simulink model "BrakeCtrl_V1"  (R2018a)
settings: Solver=VariableStepAuto  StartTime=0.0  StopTime=10.0  FixedStep=sampletime  RelTol=1e-3  EnableMultiTasking=on
PreLoadFcn:
  | BrakeCtrl_V1_PreLoad
values from neighbouring files (symbols this model uses):
  DrvReqBrkTrqMax_K = 500    [BrakeCtrl_V1_PreLoad.m]
  RegnBrkFct_K = 1.0    (= 1)    [BrakeCtrl_V1_PreLoad.m]
libraries: simulink x2
settings Model: Creator=IAEC nishito  LastModifiedBy=nishito
settings DataIOCC: LimitDataPoints=on  SaveFormat=Array  SignalLoggingSaveFormat=ModelDataLogs  SaveOutput=off  SaveTime=off
settings OptimizationCC: DefaultParameterBehavior=Inlined  ExpressionDepthLimit=2147483647  LifeSpan=inf
settings DebuggingCC: UnderspecifiedInitializationDetection=Classic  MergeDetectMultiDrivingBlocksExec=none  SolverPrmCheckMsg=warning  FcnCallInpInsideContextMsg=warning  StateNameClashWarn=warning  SFUnexpectedBacktrackingDiag=warning  SFNoUnconditionalDefaultTransitionDiag=warning  SFExecutionAtInitializationDiag=none
settings HardwareCC: ProdBitPerPointer=32  ProdBitPerSizeT=32  ProdBitPerPtrDiffT=32  ProdLargestAtomicFloat=None  ProdIntDivRoundTo=Undefined  ProdEndianess=Unspecified  ProdWordSize=32  ProdHWDeviceType=32-bit Generic
settings ModelReferenceCC: UpdateModelReferenceTargets=IfOutOfDate  PropagateSignalLabelsOutOfModel=off
settings CodeAppCC: StateflowObjectComments=on
settings GRTTargetCC: TargetLangStandard=C89/C90 (ANSI)  GeneratePreprocessorConditionals=Disable all  CombineOutputUpdateFcns=off  GRTInterface=on
settings ConfigComp: CovMetricSettings=dw  CovHtmlReporting=on  CovSaveCumulativeToWorkspaceVar=on  CovSaveSingleToWorkspaceVar=on  CovExternalEMLEnable=off

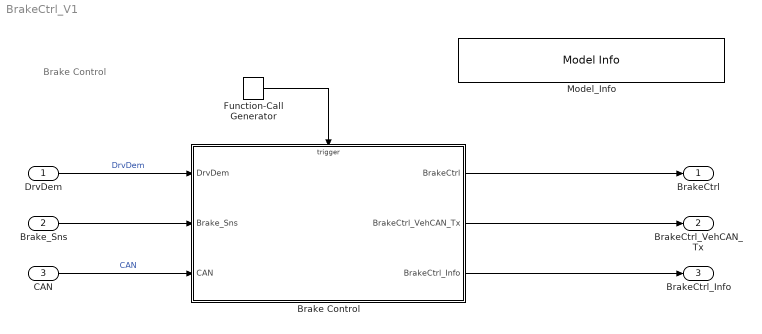
== system BrakeCtrl_V1 ==
  note: Brake Control
  DrvDem : Inport  OutDataTypeStr=Bus: Driver_demand_Bus
      settings: AttributesFormatString=%<OutDataTypeStr>
  Brake_Sns : Inport  Port=2  OutDataTypeStr=Bus: Brake_sensor_Bus
      settings: AttributesFormatString=%<OutDataTypeStr>
  CAN : Inport  Port=3  OutDataTypeStr=Bus: CAN_Bus
      settings: AttributesFormatString=<%<OutDataTypeStr>>
  Brake Control : Subsystem
  Function-Call Generator : simulink/Ports & Subsystems/Function-Call Generator  sample_time=0.01  numberOfIterations=1
      settings: AttributesFormatString=<sample_time=%<sample_time>>
  Model_Info : simulink/Model-Wide Utilities/Model Info  Frame=on  DisplayStringWithTags=|  HorizontalTextAlignment=Left  LeftAlignmentValue=0.02
      | Version  %<ModelVersion>
      | LastModifided by %<LastModifiedBy>  Date %<LastModificationDate>
      | Description  %<Description>
  BrakeCtrl : Outport  OutDataTypeStr=Bus: BrakeCtrl_Bus
      settings: AttributesFormatString=<%<OutDataTypeStr>>
  BrakeCtrl_VehCAN_Tx : Outport  Port=2  OutDataTypeStr=Bus: BrakeCtrl_VehCAN_Tx_Bus
      settings: AttributesFormatString=<%<OutDataTypeStr>>
  BrakeCtrl_Info : Outport  Port=3  OutDataTypeStr=Bus: BrakeCtrl_Info_Bus
      settings: AttributesFormatString=<%<OutDataTypeStr>>
  wires:
  CAN/1 -> Brake Control/3(CAN)  "CAN"
  DrvDem/1 -> Brake Control/1(DrvDem)  "DrvDem"
  Brake_Sns/1 -> Brake Control/2(Brake_Sns)
  Function-Call Generator/1 -> Brake Control/Trigger
  Brake Control/2(BrakeCtrl_VehCAN_Tx) -> BrakeCtrl_VehCAN_Tx/1
  Brake Control/1(BrakeCtrl) -> BrakeCtrl/1
  Brake Control/3(BrakeCtrl_Info) -> BrakeCtrl_Info/1

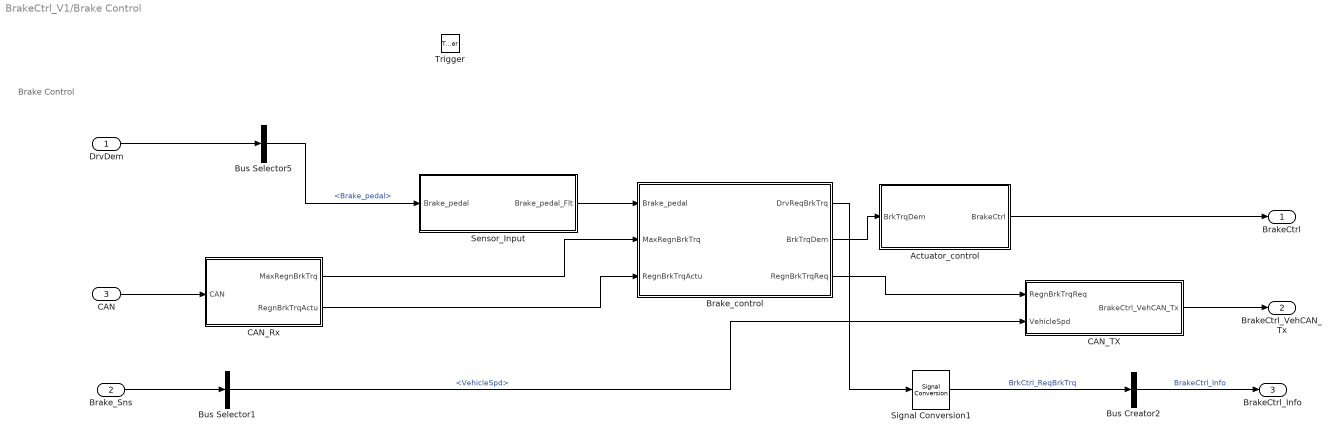
== system BrakeCtrl_V1/Brake Control ==
  note: Brake Control
  DrvDem : Inport
  Brake_Sns : Inport  Port=2
  CAN : Inport  Port=3
  Trigger : TriggerPort  TriggerType=function-call  VariantControl=Variant  PortDimensions=1
  Actuator_control : Subsystem
  Brake_control : Subsystem
  Bus Creator2 : BusCreator  Inputs=1  OutDataTypeStr=Bus: BrakeCtrl_Info_Bus
      settings: AttributesFormatString=%<OutDataTypeStr>
  Bus Selector1 : BusSelector  OutputSignals=VehicleSpd
  Bus Selector5 : BusSelector  OutputSignals=Brake_pedal
  CAN_Rx : Subsystem
  CAN_TX : Subsystem
  Sensor_Input : Subsystem
  Signal Conversion1 : SignalConversion  OverrideOpt=off
  BrakeCtrl : Outport
  BrakeCtrl_VehCAN_Tx : Outport  Port=2
  BrakeCtrl_Info : Outport  Port=3
  wires:
  Brake_Sns/1 -> Bus Selector1/1
  Bus Creator2/1 -> BrakeCtrl_Info/1  "BrakeCtrl_Info"
  Brake_control/3(RegnBrkTrqReq) -> CAN_TX/1(RegnBrkTrqReq)
  CAN_TX/1(BrakeCtrl_VehCAN_Tx) -> BrakeCtrl_VehCAN_Tx/1
  Actuator_control/1(BrakeCtrl) -> BrakeCtrl/1
  Sensor_Input/1(Brake_pedal_Flt) -> Brake_control/1(Brake_pedal)
  Brake_control/2(BrkTrqDem) -> Actuator_control/1(BrkTrqDem)
  DrvDem/1 -> Bus Selector5/1
  Bus Selector5/1 -> Sensor_Input/1(Brake_pedal)  "<Brake_pedal>"
  Bus Selector1/1 -> CAN_TX/2(VehicleSpd)  "<VehicleSpd>"
  Brake_control/1(DrvReqBrkTrq) -> Signal Conversion1/1
  CAN/1 -> CAN_Rx/1(CAN)
  CAN_Rx/1(MaxRegnBrkTrq) -> Brake_control/2(MaxRegnBrkTrq)
  CAN_Rx/2(RegnBrkTrqActu) -> Brake_control/3(RegnBrkTrqActu)
  Signal Conversion1/1 -> Bus Creator2/1  "BrkCtrl_ReqBrkTrq"

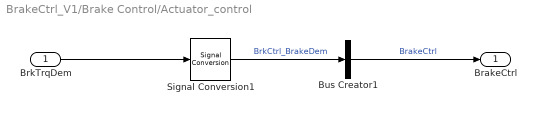
== system BrakeCtrl_V1/Brake Control/Actuator_control ==
  BrkTrqDem : Inport
  Bus Creator1 : BusCreator  Inputs=1  OutDataTypeStr=Bus: BrakeCtrl_Bus
      settings: AttributesFormatString=%<OutDataTypeStr>
  Signal Conversion1 : SignalConversion  OverrideOpt=off
  BrakeCtrl : Outport
  wires:
  Signal Conversion1/1 -> Bus Creator1/1  "BrkCtrl_BrakeDem"
  BrkTrqDem/1 -> Signal Conversion1/1
  Bus Creator1/1 -> BrakeCtrl/1  "BrakeCtrl"

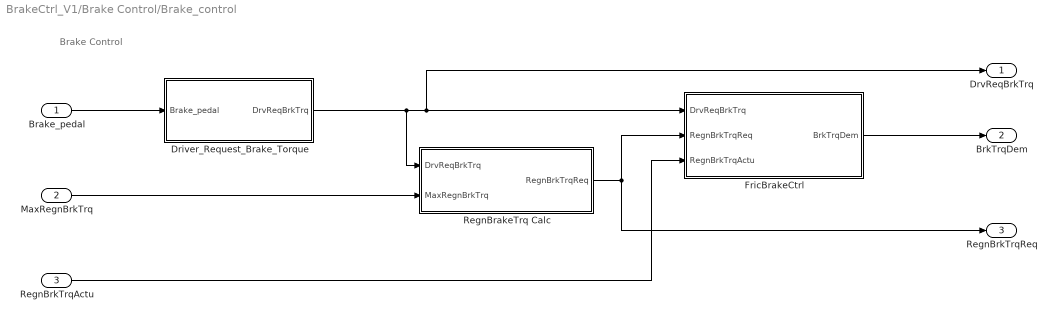
== system BrakeCtrl_V1/Brake Control/Brake_control ==
  note: Brake Control
  Brake_pedal : Inport
  MaxRegnBrkTrq : Inport  Port=2
  RegnBrkTrqActu : Inport  Port=3
  Driver_Request_Brake_Torque : Subsystem
  FricBrakeCtrl : Subsystem
  RegnBrakeTrq Calc : Subsystem
  DrvReqBrkTrq : Outport
  BrkTrqDem : Outport  Port=2
  RegnBrkTrqReq : Outport  Port=3
  wires:
  FricBrakeCtrl/1(BrkTrqDem) -> BrkTrqDem/1
  Brake_pedal/1 -> Driver_Request_Brake_Torque/1(Brake_pedal)
  MaxRegnBrkTrq/1 -> RegnBrakeTrq Calc/2(MaxRegnBrkTrq)
  RegnBrkTrqActu/1 -> FricBrakeCtrl/3(RegnBrkTrqActu)
  Driver_Request_Brake_Torque/1(DrvReqBrkTrq) -> RegnBrakeTrq Calc/1(DrvReqBrkTrq), DrvReqBrkTrq/1, FricBrakeCtrl/1(DrvReqBrkTrq)
  RegnBrakeTrq Calc/1(RegnBrkTrqReq) -> FricBrakeCtrl/2(RegnBrkTrqReq), RegnBrkTrqReq/1

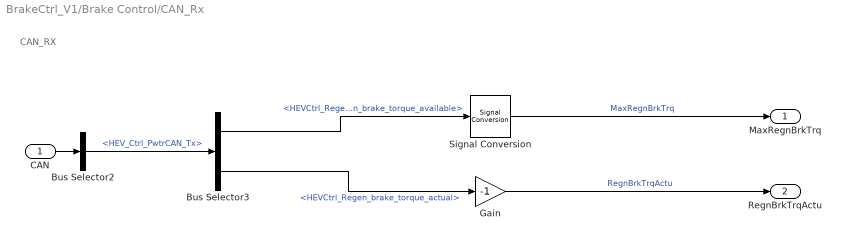
== system BrakeCtrl_V1/Brake Control/CAN_Rx ==
  note: CAN_RX
  CAN : Inport
  Bus Selector2 : BusSelector  OutputSignals=PwtrCAN.HEV_Ctrl_PwtrCAN_Tx
  Bus Selector3 : BusSelector  OutputSignals=HEVCtrl_Regen_brake_torque_available,HEVCtrl_Regen_brake_torque_actual
  Gain : Gain  Gain=-1
  Signal Conversion : SignalConversion  OverrideOpt=off
  MaxRegnBrkTrq : Outport
  RegnBrkTrqActu : Outport  Port=2
  wires:
  Bus Selector2/1 -> Bus Selector3/1  "<HEV_Ctrl_PwtrCAN_Tx>"
  CAN/1 -> Bus Selector2/1
  Gain/1 -> RegnBrkTrqActu/1  "RegnBrkTrqActu"
  Signal Conversion/1 -> MaxRegnBrkTrq/1  "MaxRegnBrkTrq"
  Bus Selector3/1 -> Signal Conversion/1  "<HEVCtrl_Regen_brake_torque_available>"
  Bus Selector3/2 -> Gain/1  "<HEVCtrl_Regen_brake_torque_actual>"

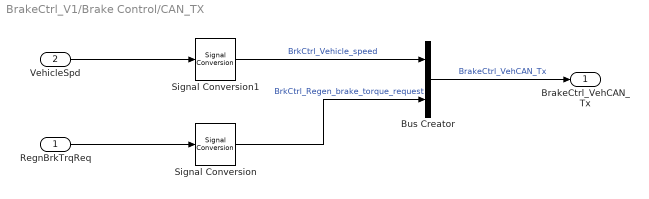
== system BrakeCtrl_V1/Brake Control/CAN_TX ==
  RegnBrkTrqReq : Inport
  VehicleSpd : Inport  Port=2
  Bus Creator : BusCreator  Inputs=2  OutDataTypeStr=Bus: BrakeCtrl_VehCAN_Tx_Bus
      settings: AttributesFormatString=%<OutDataTypeStr>
  Signal Conversion : SignalConversion  OverrideOpt=off
  Signal Conversion1 : SignalConversion  OverrideOpt=off
  BrakeCtrl_VehCAN_Tx : Outport
  wires:
  Signal Conversion/1 -> Bus Creator/2  "BrkCtrl_Regen_brake_torque_request"
  RegnBrkTrqReq/1 -> Signal Conversion/1
  Bus Creator/1 -> BrakeCtrl_VehCAN_Tx/1  "BrakeCtrl_VehCAN_Tx"
  VehicleSpd/1 -> Signal Conversion1/1
  Signal Conversion1/1 -> Bus Creator/1  "BrkCtrl_Vehicle_speed"

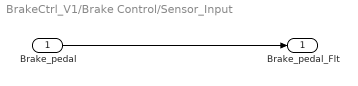
== system BrakeCtrl_V1/Brake Control/Sensor_Input ==
  Brake_pedal : Inport
  Brake_pedal_Flt : Outport
  wires:
  Brake_pedal/1 -> Brake_pedal_Flt/1

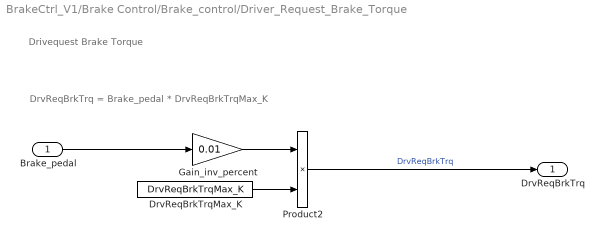
== system BrakeCtrl_V1/Brake Control/Brake_control/Driver_Request_Brake_Torque ==
  note: DrvReqBrkTrq = Brake_pedal * DrvReqBrkTrqMax_K
  note: Drivequest Brake Torque
  Brake_pedal : Inport
  DrvReqBrkTrqMax_K : Constant  Value=DrvReqBrkTrqMax_K
  Gain_inv_percent : Gain  Gain=0.01
  Product2 : Product  RndMeth=Zero
  DrvReqBrkTrq : Outport
  wires:
  Gain_inv_percent/1 -> Product2/1
  Product2/1 -> DrvReqBrkTrq/1  "DrvReqBrkTrq"
  DrvReqBrkTrqMax_K/1 -> Product2/2
  Brake_pedal/1 -> Gain_inv_percent/1

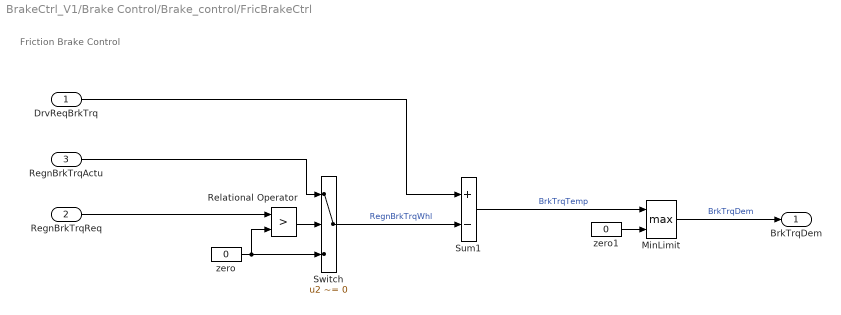
== system BrakeCtrl_V1/Brake Control/Brake_control/FricBrakeCtrl ==
  note: Friction Brake Control
  DrvReqBrkTrq : Inport
  RegnBrkTrqReq : Inport  Port=2
  RegnBrkTrqActu : Inport  Port=3
  MinLimit : MinMax  Function=max  Inputs=2
  Relational Operator : RelationalOperator  Operator=>  OutDataTypeStr=boolean  RndMeth=Nearest
  Sum1 : Sum  Inputs=+-
  Switch : Switch  Criteria=u2 ~= 0  Threshold=0.5  SaturateOnIntegerOverflow=on
      settings: AttributesFormatString=<%<Criteria>>
  zero : Constant  Value=0
  zero1 : Constant  Value=0
  BrkTrqDem : Outport
  wires:
  Switch/1 -> Sum1/2  "RegnBrkTrqWhl"
  zero/1 -> Relational Operator/2, Switch/3
  Relational Operator/1 -> Switch/2
  Sum1/1 -> MinLimit/1  "BrkTrqTemp"
  zero1/1 -> MinLimit/2
  DrvReqBrkTrq/1 -> Sum1/1
  RegnBrkTrqActu/1 -> Switch/1
  RegnBrkTrqReq/1 -> Relational Operator/1
  MinLimit/1 -> BrkTrqDem/1  "BrkTrqDem"

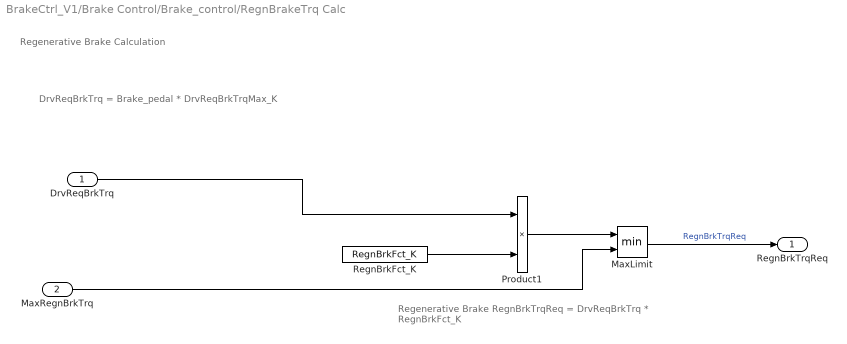
== system BrakeCtrl_V1/Brake Control/Brake_control/RegnBrakeTrq Calc ==
  note: Regenerative Brake Calculation
  note: Regenerative  Brake
      |  RegnBrkTrqReq = DrvReqBrkTrq * RegnBrkFct_K
  note: DrvReqBrkTrq = Brake_pedal * DrvReqBrkTrqMax_K
  DrvReqBrkTrq : Inport
  MaxRegnBrkTrq : Inport  Port=2
  MaxLimit : MinMax  Inputs=2
  Product1 : Product  RndMeth=Zero
  RegnBrkFct_K : Constant  Value=RegnBrkFct_K
  RegnBrkTrqReq : Outport
  wires:
  RegnBrkFct_K/1 -> Product1/2
  Product1/1 -> MaxLimit/1
  MaxRegnBrkTrq/1 -> MaxLimit/2
  MaxLimit/1 -> RegnBrkTrqReq/1  "RegnBrkTrqReq"
  DrvReqBrkTrq/1 -> Product1/1
